simulink model "single_track_3DOF"  (R2017b)
settings: Solver=ode4  StartTime=0.0  StopTime=4  FixedStep=0.001  RelTol=1e-3
settings Model: Creator=Ge Qiang  LastModifiedBy=Ge Qiang

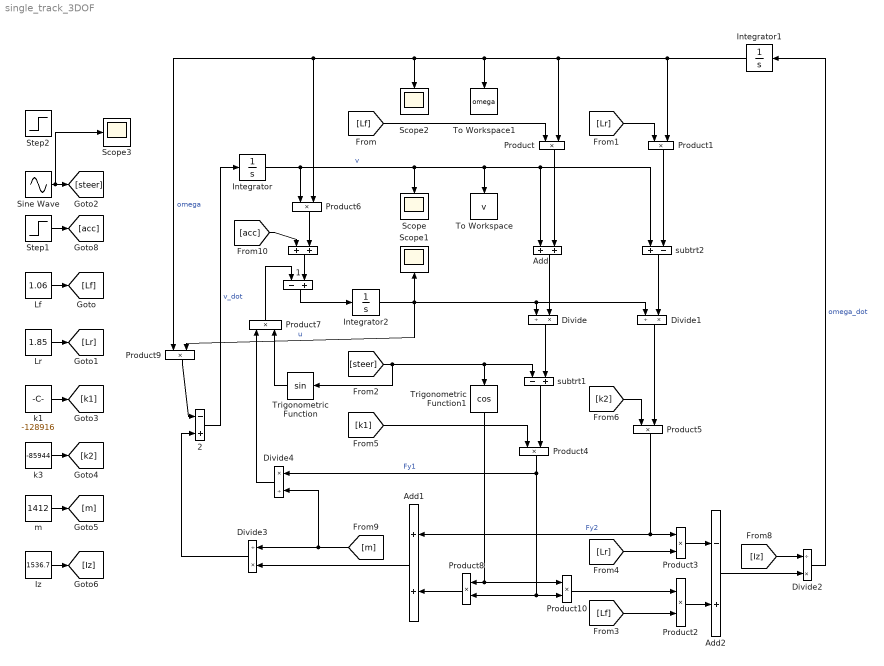
== system single_track_3DOF ==
  " " : Sum
  " 1" : Sum  Inputs=-+
  " 2" : Sum  Inputs=-+
  Add : Sum
  Add1 : Sum
  Add2 : Sum  Inputs=-+
  Divide{,1..3} (4 alike) : Product  Inputs=/*
  Divide4 : Product  Inputs=*/
  Integrator : Integrator
  Integrator1 : Integrator
  Integrator2 : Integrator  InitialCondition=8
  Iz : Constant  Value=1536.7
  Lf : Constant  Value=1.06
  Lr : Constant  Value=1.85
  Product{,1..10} (11 alike) : Product
  Scope{,1..3} (4 alike) : Scope
  Sine Wave : Sin  Amplitude=0.3  Frequency=pi  SampleTime=0
  Step1 : Step  After=0  SampleTime=0
  Step2 : Step  Time=0  After=0.2674  SampleTime=0
  To Workspace : ToWorkspace  VariableName=v  SampleTime=-1
  To Workspace1 : ToWorkspace  VariableName=omega  SampleTime=-1
  Trigonometric Function : Trigonometry
  Trigonometric Function1 : Trigonometry  Operator=cos
  k1 : Constant  Value=-128916
  k3 : Constant  Value=-85944
  m : Constant  Value=1412
  subtrt1 : Sum  Inputs=-+
  subtrt2 : Sum  Inputs=+-
  wires:
  Integrator1/1 -> Product1/2, Product/2, To Workspace1/1, Scope2/1, Product6/2, Product9/1  "omega"
  Product/1 -> Add/2
  Integrator/1 -> Product6/1, subtrt2/1, Add/1, To Workspace/1, Scope/1  "v"
  Add/1 -> Divide/2
  Sine Wave/1 -> Scope3/1, [steer]
  Product1/1 -> subtrt2/2
  Divide/1 -> subtrt1/2
  subtrt2/1 -> Divide1/2
  Divide1/1 -> Product5/2
  subtrt1/1 -> Product4/2
  Product4/1 -> Divide4/1, Product8/2, Product10/2  "Fy1"
  Product5/1 -> Product3/1, Add1/1  "Fy2"
  Add1/1 -> Divide3/2
  Divide3/1 -> " 2"/2
  Product2/1 -> Add2/2
  Product3/1 -> Add2/1
  Add2/1 -> Divide2/2
  Lf/1 -> [Lf]
  [Lf] -> Product/1
  Lr/1 -> [Lr]
  [Lr] -> Product1/1
  [steer] -> subtrt1/1, Trigonometric Function1/1, Trigonometric Function/1
  [Lf] -> Product2/2
  [Lr] -> Product3/2
  k1/1 -> [k1]
  k3/1 -> [k2]
  [k1] -> Product4/1
  [k2] -> Product5/1
  Iz/1 -> [Iz]
  m/1 -> [m]
  Integrator2/1 -> Divide1/1, Divide/1, Product9/2, Scope1/1  "u"
  [Iz] -> Divide2/1
  [m] -> Divide4/2, Divide3/1
  Step1/1 -> [acc]
  [acc] -> " "/1
  Divide2/1 -> Integrator1/1  "omega_dot"
  Product6/1 -> " "/2
  " "/1 -> " 1"/2
  Trigonometric Function/1 -> Product7/2
  Product7/1 -> " 1"/1
  Divide4/1 -> Product7/1
  " 1"/1 -> Integrator2/1
  Trigonometric Function1/1 -> Product10/1, Product8/1
  Product8/1 -> Add1/2
  Product9/1 -> " 2"/1
  " 2"/1 -> Integrator/1  "v_dot"
  Product10/1 -> Product2/1
